simulink model "vehicleID"  (R2016b)
settings: Solver=FixedStepAuto  StartTime=0.0  StopTime=600  FixedStep=1e-1
model workspace (MAT data in the model file):
  Ffun : class16 (value not decoded)
  Fnominal = 102.067398446
  Gfun : class16 (value not decoded)
  Tnominal = 0.137372003292
  deltaStep = 0.446030958824
  myVehicleModel = tf
  myVehicleModel.IOSize_ = [1 1]
  myVehicleModel.Data_ = ltipack.tfdata
  myVehicleModel.Data_.num = {[0 270]}
  myVehicleModel.Data_.den = {[100 1]}
  myVehicleModel.Data_.Delay.Input = 0
  myVehicleModel.Data_.Delay.Output = 0
  myVehicleModel.Data_.Delay.IO = 0
  myVehicleModel.Data_.Ts = 0
  tau = 0.1
  vnominal = 72.7404559749
  vnominalms = 20.2056822152
symbols that are objects in the model workspace (value not decoded): Ffun, Gfun
libraries: cstblocks x1
settings Model: Creator=jamessaunderson  LastModifiedBy=jamessaunderson
settings DataIOCC: ReturnWorkspaceOutputs=on
settings SFSimCC: SimUseLocalCustomCode=on
settings RTWCC: RTWUseLocalCustomCode=on

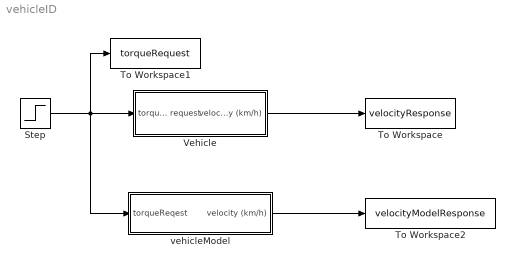
== system vehicleID ==
  Step : Step  Time=10  Before=Tnominal  After=(1+deltaStep)*Tnominal  SampleTime=0
  To Workspace : ToWorkspace  VariableName=velocityResponse  SaveFormat=Timeseries  SampleTime=-1
  To Workspace1 : ToWorkspace  VariableName=torqueRequest  SaveFormat=Timeseries  SampleTime=-1
  To Workspace2 : ToWorkspace  VariableName=velocityModelResponse  SaveFormat=Timeseries  SampleTime=-1
  Vehicle : Subsystem
  vehicleModel : Subsystem
  wires:
  Vehicle/1(velocity (km/h)) -> To Workspace/1
  Step/1 -> vehicleModel/1(torqueReqest), To Workspace1/1, Vehicle/1(torque request)
  vehicleModel/1(velocity (km/h)) -> To Workspace2/1

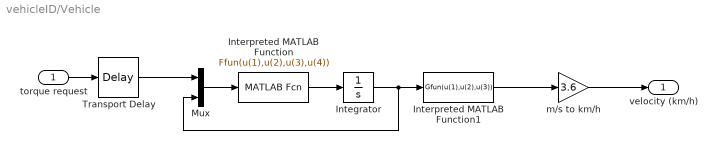
== system vehicleID/Vehicle ==
  torque request : Inport
  Integrator : Integrator  InitialCondition=[0;vnominalms;Fnominal]
  Interpreted MATLAB Function : MATLABFcn  MATLABFcn=Ffun(u(1),u(2),u(3),u(4))  OutputDimensions=3
  Interpreted MATLAB Function1 : MATLABFcn  MATLABFcn=Gfun(u(1),u(2),u(3))  OutputDimensions=1
  Mux : Mux  Inputs=2
  Transport Delay : TransportDelay  DelayTime=tau  InitialOutput=Tnominal
  m/s to km/h : Gain  Gain=3.6
  velocity (km/h) : Outport
  wires:
  Transport Delay/1 -> Mux/1
  torque request/1 -> Transport Delay/1
  Interpreted MATLAB Function/1 -> Integrator/1
  Integrator/1 -> Mux/2, Interpreted MATLAB Function1/1
  Mux/1 -> Interpreted MATLAB Function/1
  Interpreted MATLAB Function1/1 -> m/s to km/h/1
  m/s to km/h/1 -> velocity (km/h)/1

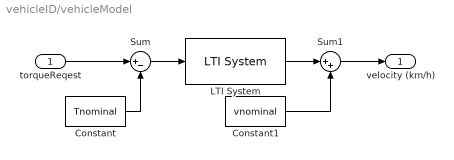
== system vehicleID/vehicleModel ==
  torqueReqest : Inport
  Constant : Constant  Value=Tnominal
  Constant1 : Constant  Value=vnominal
  LTI System : cstblocks/LTI System  sys=myVehicleModel  IC=[]
  Sum : Sum  Inputs=|+-
  Sum1 : Sum  Inputs=|++
  velocity (km/h) : Outport
  wires:
  Sum1/1 -> velocity (km/h)/1
  Constant1/1 -> Sum1/2
  Sum/1 -> LTI System/1
  LTI System/1 -> Sum1/1
  Constant/1 -> Sum/2
  torqueReqest/1 -> Sum/1
